simulink library "Blocks_Lib"  (R2019b)
settings: Solver=VariableStepAuto  StartTime=0.0  StopTime=10.0  RelTol=1e-3
libraries: simulink x9, $bdroot x9
(part 2 of 2)

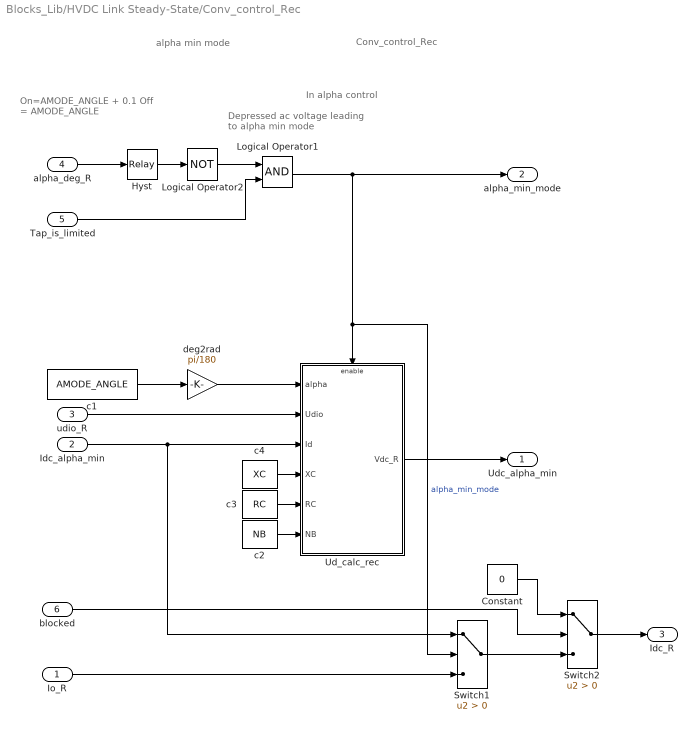
== system Blocks_Lib/HVDC Link Steady-State/Conv_control_Rec ==
  note: Depressed ac voltage
      |  leading to alpha min mode
  note: In alpha control
  note: Conv_control_Rec
  note: On=AMODE_ANGLE + 0.1
      | Off = AMODE_ANGLE
  note: alpha min mode
  Io_R : Inport
  Idc_alpha_min : Inport  Port=2
  udio_R : Inport  Port=3
  alpha_deg_R : Inport  Port=4
  Tap_is_limited : Inport  Port=5
  blocked : Inport  Port=6
  Constant : Constant  Value=0
  Hyst : Relay  OnSwitchValue=AMODE_ANGLE + 0.1  OffSwitchValue=AMODE_ANGLE
  Logical Operator1 : Logic  AllPortsSameDT=off  OutDataTypeStr=boolean
  Logical Operator2 : Logic  Operator=NOT  AllPortsSameDT=off  OutDataTypeStr=boolean
  Switch1 : Switch  Criteria=u2 > Threshold
  Switch2 : Switch  Criteria=u2 > Threshold
  Ud_calc_rec : Subsystem
  c1 : Constant  Value=AMODE_ANGLE
  c2 : Constant  Value=NB
  c3 : Constant  Value=RC
  c4 : Constant  Value=XC
  "deg2rad " : Gain  Gain=pi/180
  Udc_alpha_min : Outport
  alpha_min_mode : Outport  Port=2
  Idc_R : Outport  Port=3
  wires:
  Tap_is_limited/1 -> Logical Operator1/2
  Io_R/1 -> Switch1/3
  Logical Operator1/1 -> alpha_min_mode/1, Ud_calc_rec/Enable, Switch1/2  "alpha_min_mode"
  "deg2rad "/1 -> Ud_calc_rec/1(alpha)
  c1/1 -> "deg2rad "/1
  udio_R/1 -> Ud_calc_rec/2(Udio)
  c3/1 -> Ud_calc_rec/5(RC)
  c4/1 -> Ud_calc_rec/4(XC)
  alpha_deg_R/1 -> Hyst/1
  Ud_calc_rec/1(Vdc_R) -> Udc_alpha_min/1
  Idc_alpha_min/1 -> Ud_calc_rec/3(Id), Switch1/1
  Switch1/1 -> Switch2/3
  Switch2/1 -> Idc_R/1
  Constant/1 -> Switch2/1
  blocked/1 -> Switch2/2
  Hyst/1 -> Logical Operator2/1
  Logical Operator2/1 -> Logical Operator1/1
  c2/1 -> Ud_calc_rec/6(NB)

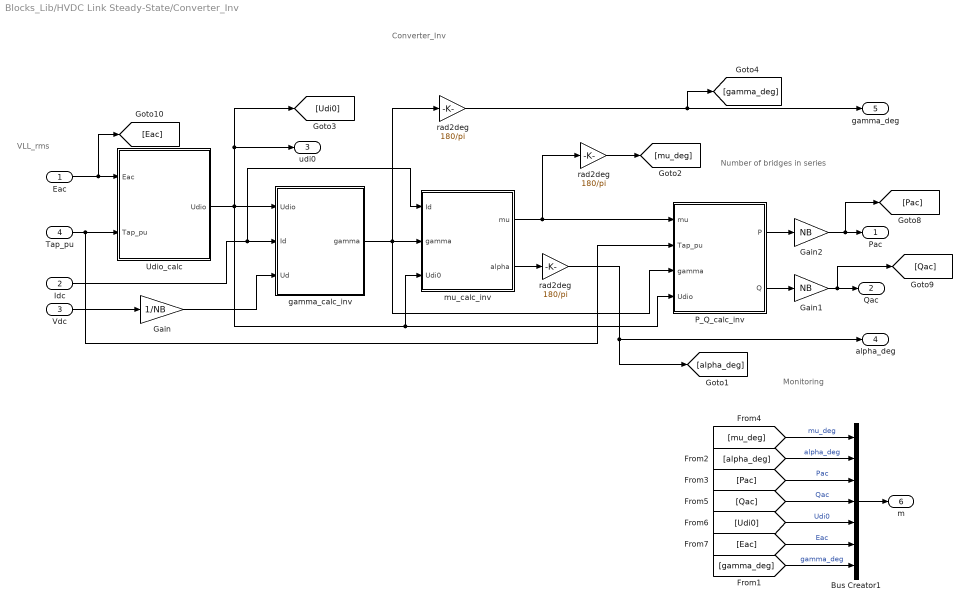
== system Blocks_Lib/HVDC Link Steady-State/Converter_Inv ==
  note: Monitoring
  note: Number of bridges in series
  note: VLL_rms
  note: Converter_Inv
  Eac : Inport
  Idc : Inport  Port=2
  Vdc : Inport  Port=3
  Tap_pu : Inport  Port=4
  Bus Creator1 : BusCreator  Inputs=7
  Gain : Gain  Gain=1/NB
  Gain1 : Gain  Gain=NB
  Gain2 : Gain  Gain=NB
  P_Q_calc_inv : Subsystem
  Udio_calc : Subsystem
  gamma_calc_inv : Subsystem
  mu_calc_inv : Subsystem
  "rad2deg " : Gain  Gain=180/pi
  "rad2deg  " : Gain  Gain=180/pi
  "rad2deg   " : Gain  Gain=180/pi
  Pac : Outport
  Qac : Outport  Port=2
  udi0 : Outport  Port=3
  alpha_deg : Outport  Port=4
  gamma_deg : Outport  Port=5
  m : Outport  Port=6
  wires:
  [Eac] -> Bus Creator1/6  "Eac"
  [gamma_deg] -> Bus Creator1/7  "gamma_deg"
  [Udi0] -> Bus Creator1/5  "Udi0"
  [Qac] -> Bus Creator1/4  "Qac"
  [Pac] -> Bus Creator1/3  "Pac"
  [alpha_deg] -> Bus Creator1/2  "alpha_deg"
  [mu_deg] -> Bus Creator1/1  "mu_deg"
  Bus Creator1/1 -> m/1
  "rad2deg   "/1 -> [alpha_deg], alpha_deg/1
  mu_calc_inv/2(alpha) -> "rad2deg   "/1
  mu_calc_inv/1(mu) -> "rad2deg  "/1, P_Q_calc_inv/1(mu)
  "rad2deg  "/1 -> [mu_deg]
  Gain1/1 -> [Qac], Qac/1
  Gain2/1 -> [Pac], Pac/1
  Gain/1 -> gamma_calc_inv/3(Ud)
  P_Q_calc_inv/1(P) -> Gain2/1
  P_Q_calc_inv/2(Q) -> Gain1/1
  "rad2deg "/1 -> [gamma_deg], gamma_deg/1
  gamma_calc_inv/1(gamma) -> P_Q_calc_inv/3(gamma), mu_calc_inv/2(gamma), "rad2deg "/1
  Vdc/1 -> Gain/1
  Idc/1 -> mu_calc_inv/1(Id), gamma_calc_inv/2(Id)
  Eac/1 -> [Eac], Udio_calc/1(Eac)
  Udio_calc/1(Udio) -> [Udi0], udi0/1, P_Q_calc_inv/4(Udio), mu_calc_inv/3(Udi0), gamma_calc_inv/1(Udio)
  Tap_pu/1 -> P_Q_calc_inv/2(Tap_pu), Udio_calc/2(Tap_pu)

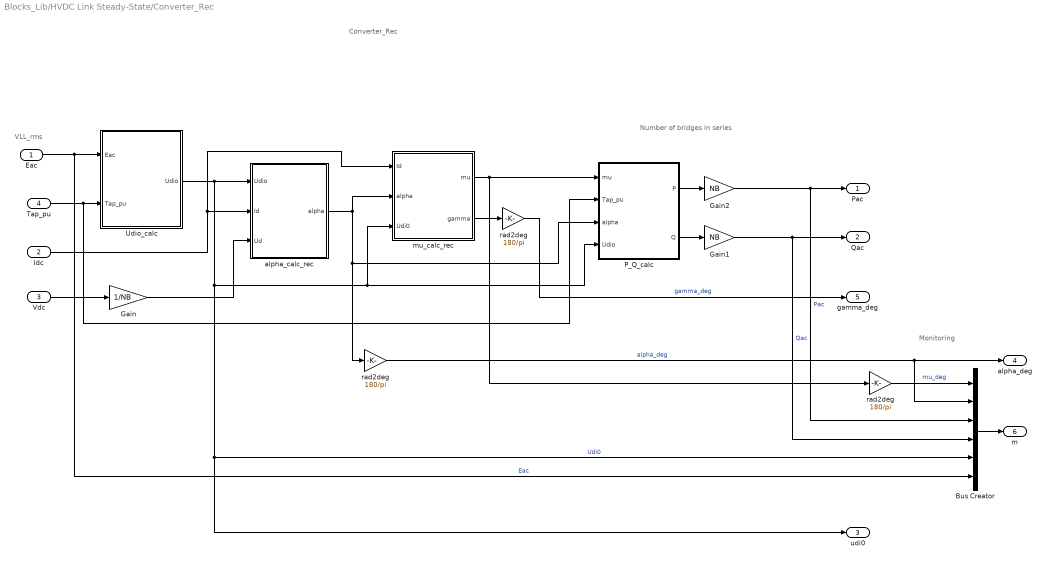
== system Blocks_Lib/HVDC Link Steady-State/Converter_Rec ==
  note: Converter_Rec
  note: VLL_rms
  note: Number of bridges in series
  note: Monitoring
  Eac : Inport
  Idc : Inport  Port=2
  Vdc : Inport  Port=3
  Tap_pu : Inport  Port=4
  Bus Creator : BusCreator  Inputs=6
  Gain : Gain  Gain=1/NB
  Gain1 : Gain  Gain=NB
  Gain2 : Gain  Gain=NB
  P_Q_calc : Subsystem
  Udio_calc : Subsystem
  alpha_calc_rec : Subsystem
  mu_calc_rec : Subsystem
  "rad2deg " : Gain  Gain=180/pi
  "rad2deg  " : Gain  Gain=180/pi
  "rad2deg   " : Gain  Gain=180/pi
  Pac : Outport
  Qac : Outport  Port=2
  udi0 : Outport  Port=3
  alpha_deg : Outport  Port=4
  gamma_deg : Outport  Port=5
  m : Outport  Port=6
  wires:
  Eac/1 -> Udio_calc/1(Eac), Bus Creator/6  "Eac"
  Udio_calc/1(Udio) -> udi0/1, Bus Creator/5, mu_calc_rec/3(Udi0), P_Q_calc/4(Udio), alpha_calc_rec/1(Udio)  "Udi0"
  Gain1/1 -> Bus Creator/4, Qac/1  "Qac"
  Gain2/1 -> Bus Creator/3, Pac/1  "Pac"
  "rad2deg "/1 -> Bus Creator/2, alpha_deg/1  "alpha_deg"
  "rad2deg  "/1 -> Bus Creator/1  "mu_deg"
  Tap_pu/1 -> P_Q_calc/2(Tap_pu), Udio_calc/2(Tap_pu)
  Idc/1 -> alpha_calc_rec/2(Id), mu_calc_rec/1(Id)
  Vdc/1 -> Gain/1
  alpha_calc_rec/1(alpha) -> "rad2deg "/1, P_Q_calc/3(alpha), mu_calc_rec/2(alpha)
  mu_calc_rec/1(mu) -> P_Q_calc/1(mu), "rad2deg  "/1
  mu_calc_rec/2(gamma) -> "rad2deg   "/1
  P_Q_calc/2(Q) -> Gain1/1
  P_Q_calc/1(P) -> Gain2/1
  Gain/1 -> alpha_calc_rec/3(Ud)
  Bus Creator/1 -> m/1
  "rad2deg   "/1 -> gamma_deg/1  "gamma_deg"

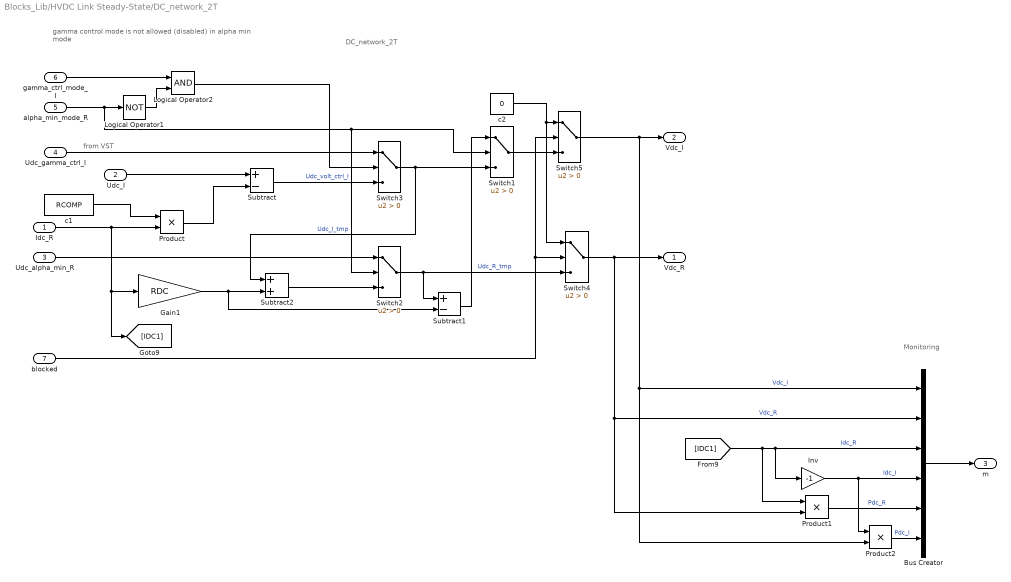
== system Blocks_Lib/HVDC Link Steady-State/DC_network_2T ==
  note: gamma control mode is not allowed (disabled)
      |  in alpha min mode
  note: DC_network_2T
  note: Monitoring
  note: from VST
  Idc_R : Inport
  Udc_I : Inport  Port=2
  Udc_alpha_min_R : Inport  Port=3
  Udc_gamma_ctrl_I : Inport  Port=4
  alpha_min_mode_R : Inport  Port=5
  gamma_ctrl_mode_I : Inport  Port=6
  blocked : Inport  Port=7
  Bus Creator : BusCreator  Inputs=6
  Gain1 : Gain  Gain=RDC
  Inv : Gain  Gain=-1
  Logical Operator1 : Logic  Operator=NOT  AllPortsSameDT=off  OutDataTypeStr=boolean
  Logical Operator2 : Logic  AllPortsSameDT=off  OutDataTypeStr=boolean
  Product : Product  RndMeth=Zero
  Product1 : Product  RndMeth=Zero
  Product2 : Product  RndMeth=Zero
  Subtract : Sum  Inputs=+-
  Subtract1 : Sum  Inputs=+-
  Subtract2 : Sum
  Switch{1..5} (5 alike) : Switch  Criteria=u2 > Threshold
  c1 : Constant  Value=RCOMP
  c2 : Constant  Value=0
  Vdc_R : Outport
  Vdc_I : Outport  Port=2
  m : Outport  Port=3
  wires:
  Product2/1 -> Bus Creator/6  "Pdc_I"
  [IDC1] -> Bus Creator/3, Inv/1, Product1/1  "Idc_R"
  Product1/1 -> Bus Creator/5  "Pdc_R"
  Inv/1 -> Product2/1, Bus Creator/4  "Idc_I"
  Logical Operator2/1 -> Switch3/2
  alpha_min_mode_R/1 -> Switch1/2, Switch2/2, Logical Operator1/1
  Logical Operator1/1 -> Logical Operator2/2
  gamma_ctrl_mode_I/1 -> Logical Operator2/1
  Udc_I/1 -> Subtract/1
  Idc_R/1 -> [IDC1], Gain1/1, Product/2
  Subtract/1 -> Switch3/3  "Udc_volt_ctrl_I"
  Udc_gamma_ctrl_I/1 -> Switch3/1
  Switch3/1 -> Switch1/3, Subtract2/1  "Udc_I_tmp"
  Gain1/1 -> Subtract2/2, Subtract1/2
  Subtract2/1 -> Switch2/3
  Udc_alpha_min_R/1 -> Switch2/1
  Switch2/1 -> Subtract1/1, Switch4/3  "Udc_R_tmp"
  Subtract1/1 -> Switch1/1
  Product/1 -> Subtract/2
  c1/1 -> Product/1
  Bus Creator/1 -> m/1
  Switch5/1 -> Bus Creator/1, Product2/2, Vdc_I/1  "Vdc_I"
  Switch4/1 -> Bus Creator/2, Product1/2, Vdc_R/1  "Vdc_R"
  Switch1/1 -> Switch5/3
  blocked/1 -> Switch4/2, Switch5/2
  c2/1 -> Switch5/1, Switch4/1

== system Blocks_Lib/HVDC Link Steady-State/LF_Soution_Criteria ==
  note: convergence criteria for DC LF solution
  Tap_R : Inport
  Tap_I : Inport  Port=2
  Tap_is_limited_R : Inport  Port=3
  Tap_is_limited_I : Inport  Port=4
  Abs : Abs
  Abs1 : Abs
  Compare To Constant : simulink/Logic and Bit Operations/Compare To Constant  relop=<=  const=1e-6  OutDataTypeStr=uint8
  Compare To Constant1 : simulink/Logic and Bit Operations/Compare To Constant  relop=<=  const=1e-6  OutDataTypeStr=uint8
  Difference : simulink/Discrete/Difference  ICPrevInput=0.0  InputProcessing=Inherited  OutMin=[]  OutMax=[]  OutDataType=fixdt(1, 16)  OutScaling=2^-10  DoSatur=off
  Difference1 : simulink/Discrete/Difference  ICPrevInput=0.0  InputProcessing=Inherited  OutMin=[]  OutMax=[]  OutDataType=fixdt(1, 16)  OutScaling=2^-10  DoSatur=off
  Logical Operator : Logic  AllPortsSameDT=off  OutDataTypeStr=boolean
  Logical Operator1 : Logic  AllPortsSameDT=off  OutDataTypeStr=boolean
  Logical Operator2 : Logic  Operator=NOT  AllPortsSameDT=off  OutDataTypeStr=boolean
  Logical Operator3 : Logic  Operator=OR  AllPortsSameDT=off  OutDataTypeStr=boolean
  Logical Operator4 : Logic  AllPortsSameDT=off  OutDataTypeStr=boolean
  Logical Operator5 : Logic  Operator=OR  AllPortsSameDT=off  OutDataTypeStr=boolean
  Logical Operator6 : Logic  Operator=NOT  AllPortsSameDT=off  OutDataTypeStr=boolean
  Unit Delay1 : UnitDelay  SampleTime=-1  HasFrameUpgradeWarning=on
  Unit Delay2 : UnitDelay  SampleTime=-1  HasFrameUpgradeWarning=on
  converge : Outport
  wires:
  Tap_I/1 -> Difference/1
  Tap_R/1 -> Difference1/1
  Difference1/1 -> Abs1/1
  Abs1/1 -> Compare To Constant1/1
  Abs/1 -> Compare To Constant/1
  Logical Operator/1 -> converge/1
  Difference/1 -> Abs/1
  Compare To Constant/1 -> Logical Operator1/1
  Tap_is_limited_I/1 -> Logical Operator2/1, Unit Delay2/1
  Logical Operator2/1 -> Logical Operator1/2
  Logical Operator1/1 -> Logical Operator3/1
  Logical Operator3/1 -> Logical Operator/2
  Unit Delay2/1 -> Logical Operator3/2
  Compare To Constant1/1 -> Logical Operator4/1
  Logical Operator4/1 -> Logical Operator5/1
  Tap_is_limited_R/1 -> Unit Delay1/1, Logical Operator6/1
  Logical Operator6/1 -> Logical Operator4/2
  Unit Delay1/1 -> Logical Operator5/2
  Logical Operator5/1 -> Logical Operator/1

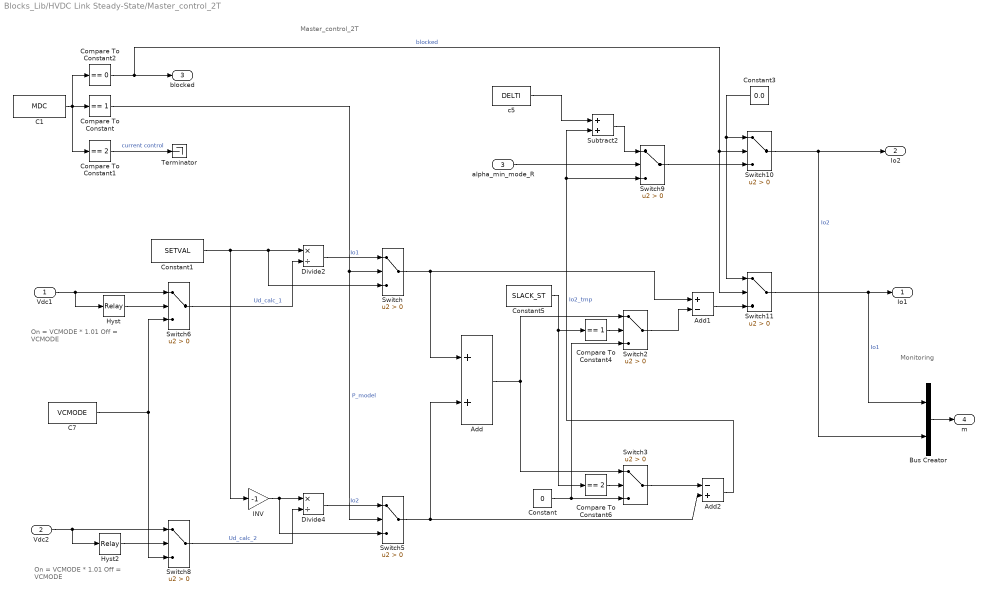
== system Blocks_Lib/HVDC Link Steady-State/Master_control_2T ==
  note: Master_control_2T
  note: On = VCMODE  * 1.01
      | Off = VCMODE
  note: On = VCMODE  * 1.01
      | Off = VCMODE
  note: Monitoring
  Vdc1 : Inport
  Vdc2 : Inport  Port=2
  alpha_min_mode_R : Inport  Port=3
  Add : Sum
  Add1 : Sum  Inputs=+-
  Add2 : Sum  Inputs=-+
  Bus Creator : BusCreator  Inputs=2
  C1 : Constant  Value=MDC
  C7 : Constant  Value=VCMODE
  Compare To Constant : simulink/Logic and Bit Operations/Compare To Constant  relop===  const=1  OutDataTypeStr=uint8  ZeroCross=off
  Compare To Constant1 : simulink/Logic and Bit Operations/Compare To Constant  relop===  const=2  OutDataTypeStr=uint8  ZeroCross=off
  Compare To Constant2 : simulink/Logic and Bit Operations/Compare To Constant  relop===  const=0  OutDataTypeStr=uint8  ZeroCross=off
  Compare To Constant4 : simulink/Logic and Bit Operations/Compare To Constant  relop===  const=1  OutDataTypeStr=uint8
  Compare To Constant6 : simulink/Logic and Bit Operations/Compare To Constant  relop===  const=2  OutDataTypeStr=uint8
  Constant : Constant  Value=0
  Constant1 : Constant  Value=SETVAL
  Constant3 : Constant  Value=0.0
  Constant5 : Constant  Value=SLACK_ST
  Divide2 : Product  Inputs=*/
  Divide4 : Product  Inputs=*/
  Hyst : Relay  OnSwitchValue=VCMODE*1.01  OffSwitchValue=VCMODE
  Hyst2 : Relay  OnSwitchValue=VCMODE*1.01  OffSwitchValue=VCMODE
  INV : Gain  Gain=-1
  Subtract2 : Sum
  Switch{,2..3,5..6,8..11} (9 alike) : Switch  Criteria=u2 > Threshold
  Terminator : Terminator
  c5 : Constant  Value=DELTI
  Io1 : Outport
  Io2 : Outport  Port=2
  blocked : Outport  Port=3
  m : Outport  Port=4
  wires:
  Switch10/1 -> Bus Creator/2, Io2/1  "Io2"
  Add1/1 -> Switch11/3
  Constant3/1 -> Switch11/1, Switch10/1
  Switch9/1 -> Switch10/3
  alpha_min_mode_R/1 -> Switch9/2
  Compare To Constant2/1 -> Switch11/2, Switch10/2, blocked/1  "blocked"
  C1/1 -> Compare To Constant1/1, Compare To Constant/1, Compare To Constant2/1
  Compare To Constant1/1 -> Terminator/1  "current control"
  Add/1 -> Switch2/1, Switch3/1
  Switch2/1 -> Add1/2
  INV/1 -> Divide4/1, Switch5/3
  Constant1/1 -> Divide2/1, Switch/3, INV/1
  Compare To Constant4/1 -> Switch2/2
  Compare To Constant6/1 -> Switch3/2
  Constant/1 -> Switch2/3, Switch3/3
  Constant5/1 -> Compare To Constant6/1, Compare To Constant4/1
  Divide2/1 -> Switch/1  "Io1"
  Divide4/1 -> Switch5/1  "Io2"
  Switch/1 -> Add/1, Add1/1
  Switch5/1 -> Add2/2, Add/2
  Compare To Constant/1 -> Switch/2, Switch5/2  "P_model"
  Switch3/1 -> Add2/1
  Hyst/1 -> Switch6/2
  C7/1 -> Switch6/3, Switch8/3
  Vdc1/1 -> Switch6/1, Hyst/1
  Hyst2/1 -> Switch8/2
  Vdc2/1 -> Switch8/1, Hyst2/1
  Switch6/1 -> Divide2/2  "Ud_calc_1"
  Switch8/1 -> Divide4/2  "Ud_calc_2"
  Bus Creator/1 -> m/1
  Add2/1 -> Subtract2/2, Switch9/3  "Io2_tmp"
  c5/1 -> Subtract2/1
  Subtract2/1 -> Switch9/1
  Switch11/1 -> Bus Creator/1, Io1/1  "Io1"

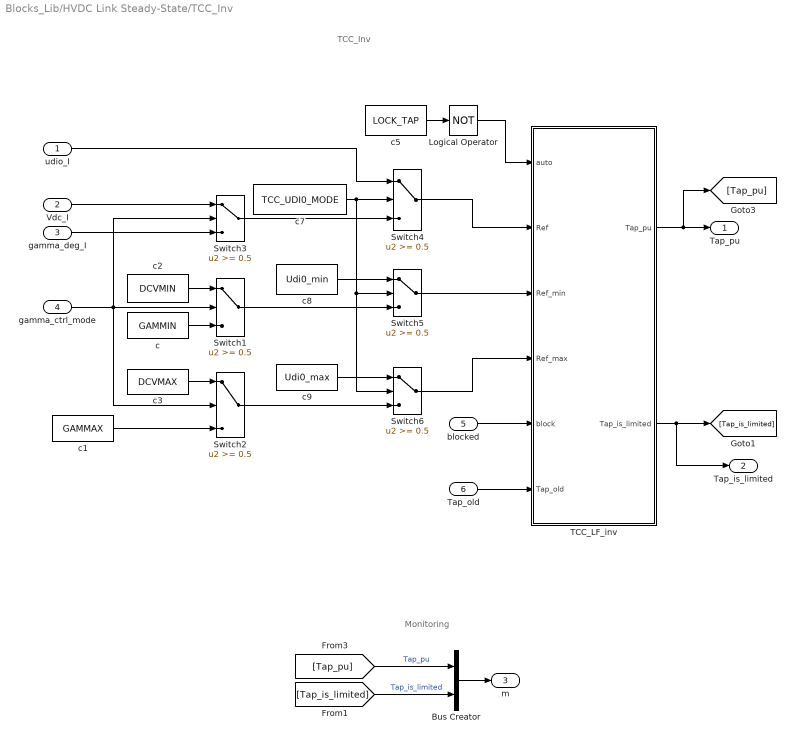
== system Blocks_Lib/HVDC Link Steady-State/TCC_Inv ==
  note: Monitoring
  note: TCC_Inv
  udio_I : Inport
  Vdc_I : Inport  Port=2
  gamma_deg_I : Inport  Port=3
  gamma_ctrl_mode : Inport  Port=4
  blocked : Inport  Port=5
  Tap_old : Inport  Port=6
  Bus Creator : BusCreator  Inputs=2
  Logical Operator : Logic  Operator=NOT  AllPortsSameDT=off  OutDataTypeStr=boolean
  Switch{1..6} (6 alike) : Switch  Threshold=0.5
  TCC_LF_inv : Subsystem
  c : Constant  Value=GAMMIN
  c1 : Constant  Value=GAMMAX
  c2 : Constant  Value=DCVMIN
  c3 : Constant  Value=DCVMAX
  c5 : Constant  Value=LOCK_TAP
  c7 : Constant  Value=TCC_UDI0_MODE
  c8 : Constant  Value=Udi0_min
  c9 : Constant  Value=Udi0_max
  Tap_pu : Outport
  Tap_is_limited : Outport  Port=2
  m : Outport  Port=3
  wires:
  [Tap_is_limited] -> Bus Creator/2  "Tap_is_limited"
  [Tap_pu] -> Bus Creator/1  "Tap_pu"
  Bus Creator/1 -> m/1
  Vdc_I/1 -> Switch3/1
  c2/1 -> Switch1/1
  c3/1 -> Switch2/1
  gamma_deg_I/1 -> Switch3/3
  c1/1 -> Switch2/3
  c/1 -> Switch1/3
  gamma_ctrl_mode/1 -> Switch3/2, Switch2/2, Switch1/2
  blocked/1 -> TCC_LF_inv/5(block)
  c5/1 -> Logical Operator/1
  Logical Operator/1 -> TCC_LF_inv/1(auto)
  udio_I/1 -> Switch4/1
  c7/1 -> Switch4/2, Switch5/2, Switch6/2
  c8/1 -> Switch5/1
  c9/1 -> Switch6/1
  Switch3/1 -> Switch4/3
  Switch1/1 -> Switch5/3
  Switch2/1 -> Switch6/3
  Switch4/1 -> TCC_LF_inv/2(Ref)
  Switch5/1 -> TCC_LF_inv/3(Ref_min)
  Switch6/1 -> TCC_LF_inv/4(Ref_max)
  Tap_old/1 -> TCC_LF_inv/6(Tap_old)
  TCC_LF_inv/2(Tap_is_limited) -> [Tap_is_limited], Tap_is_limited/1
  TCC_LF_inv/1(Tap_pu) -> [Tap_pu], Tap_pu/1

== system Blocks_Lib/HVDC Link Steady-State/TCC_Rec ==
  note: TCC_Rec
  note: Monitoring
  udio_R : Inport
  alpha_deg_R : Inport  Port=2
  blocked : Inport  Port=3
  Tap_old : Inport  Port=4
  Bus Creator : BusCreator  Inputs=2
  Logical Operator : Logic  Operator=NOT  AllPortsSameDT=off  OutDataTypeStr=boolean
  Switch4 : Switch  Threshold=0.5
  Switch5 : Switch  Threshold=0.5
  Switch6 : Switch  Threshold=0.5
  TCC_LF : Subsystem
  c1 : Constant  Value=ALFMAX
  c2 : Constant  Value=ALFMIN
  c5 : Constant  Value=LOCK_TAP
  c7 : Constant  Value=TCC_UDI0_MODE
  c8 : Constant  Value=Udi0_min
  c9 : Constant  Value=Udi0_max
  Tap_pu : Outport
  Tap_is_limited : Outport  Port=2
  m : Outport  Port=3
  wires:
  Tap_old/1 -> TCC_LF/6(Tap_old)
  blocked/1 -> TCC_LF/5(block)
  c5/1 -> Logical Operator/1
  Logical Operator/1 -> TCC_LF/1(auto)
  udio_R/1 -> Switch4/1
  c7/1 -> Switch6/2, Switch5/2, Switch4/2
  c8/1 -> Switch5/1
  c9/1 -> Switch6/1
  alpha_deg_R/1 -> Switch4/3
  c1/1 -> Switch6/3
  Switch4/1 -> TCC_LF/2(Ref)
  Switch5/1 -> TCC_LF/3(Ref_min)
  Switch6/1 -> TCC_LF/4(Ref_max)
  c2/1 -> Switch5/3
  Bus Creator/1 -> m/1
  TCC_LF/1(Tap_pu) -> Bus Creator/1, Tap_pu/1  "Tap_pu"
  TCC_LF/2(Tap_is_limited) -> Bus Creator/2, Tap_is_limited/1  "Tap_is_limited"

== system Blocks_Lib/HVDC Link Steady-State/Conv_control_Inv_vst/Ud_calc_inv ==
  note: Equivalent commtating resistance
  note: 3/pi
  note: Udio * cos(gamma)
  note: Ud_calc_inv
  note: Transformer windings & Thyristor
      |  resistance drop
  gamma : Inport
  Udio : Inport  Port=2
  Id : Inport  Port=3
  XC : Inport  Port=4
  RC : Inport  Port=5
  NB : Inport  Port=6
  Enable (held) : EnablePort  PropagateVarSize=During execution
  Gain1 : Gain  Gain=2
  Gain2 : Gain  Gain=3/pi
  Product{1..4} (4 alike) : Product  RndMeth=Zero
  Subtract : Sum  Inputs=+-+
  Trigonometric Function : Trigonometry  Operator=cos
  Vdc_I : Outport
  wires:
  gamma/1 -> Trigonometric Function/1
  Trigonometric Function/1 -> Product1/2
  Udio/1 -> Product1/1
  Product1/1 -> Subtract/1  "udio_cos_gamma"
  Id/1 -> Product2/1, Product4/1
  Product2/1 -> Subtract/2  "RcId"
  Gain2/1 -> Product2/2
  RC/1 -> Gain1/1
  Gain1/1 -> Product4/2
  Product4/1 -> Subtract/3
  XC/1 -> Gain2/1
  Subtract/1 -> Product3/1
  Product3/1 -> Vdc_I/1
  NB/1 -> Product3/2

== system Blocks_Lib/HVDC Link Steady-State/Conv_control_Rec/Ud_calc_rec ==
  note: Equivalent commtating resistance
  note: 3/pi
  note: Udio * cos(alpha)
  note: Ud_calc_rec
  note: Transformer windings & Thyristor
      |  resistance drop
  alpha : Inport
  Udio : Inport  Port=2
  Id : Inport  Port=3
  XC : Inport  Port=4
  RC : Inport  Port=5
  NB : Inport  Port=6
  Enable (held) : EnablePort  PropagateVarSize=During execution
  Gain1 : Gain  Gain=2
  Gain2 : Gain  Gain=3/pi
  Product{1..4} (4 alike) : Product  RndMeth=Zero
  Subtract : Sum  Inputs=+--
  Trigonometric Function : Trigonometry  Operator=cos
  Vdc_R : Outport
  wires:
  alpha/1 -> Trigonometric Function/1
  Trigonometric Function/1 -> Product1/2
  Udio/1 -> Product1/1
  Product1/1 -> Subtract/1  "udio_cos_alpha"
  Id/1 -> Product2/1, Product4/1
  Product2/1 -> Subtract/2  "RcId"
  Gain2/1 -> Product2/2
  RC/1 -> Gain1/1
  Gain1/1 -> Product4/2
  Product4/1 -> Subtract/3
  XC/1 -> Gain2/1
  Subtract/1 -> Product3/1
  Product3/1 -> Vdc_R/1
  NB/1 -> Product3/2

== system Blocks_Lib/HVDC Link Steady-State/Converter_Inv/P_Q_calc_inv ==
  note: Negative in inverter
      |  (gamma)
  mu : Inport
  Tap_pu : Inport  Port=2
  gamma : Inport  Port=3
  Udio : Inport  Port=4
  "Avoid zero " : Saturate  UpperLimit=inf  LowerLimit=eps
  Gain1 : Gain  Gain=NB
  Gain2 : Gain  Gain=NB
  Gain3 : Gain  Gain=-1
  Id_Iq_Pq_calc : Subsystem
  Terminator : Terminator
  Terminator1 : Terminator
  P : Outport
  Q : Outport  Port=2
  wires:
  Gain1/1 -> Terminator1/1
  Gain2/1 -> Terminator/1
  Id_Iq_Pq_calc/4(P_q) -> Q/1
  Id_Iq_Pq_calc/3(P_d) -> Gain3/1
  Udio/1 -> Id_Iq_Pq_calc/1(Udio)
  "Avoid zero "/1 -> Id_Iq_Pq_calc/2(Tap_pu)
  Tap_pu/1 -> "Avoid zero "/1
  mu/1 -> Id_Iq_Pq_calc/3(mu)
  gamma/1 -> Id_Iq_Pq_calc/4(angle)
  Id_Iq_Pq_calc/1(I_d) -> Gain2/1
  Id_Iq_Pq_calc/2(I_q) -> Gain1/1
  Gain3/1 -> P/1

== system Blocks_Lib/HVDC Link Steady-State/Converter_Inv/Udio_calc ==
  note: Udio_calc
  note: 3*sqrt(2)/pi * Usec_nom/Uprim_nom
  note: VLL_rms
  Eac : Inport
  Tap_pu : Inport  Port=2
  "Avoid zero " : Saturate  UpperLimit=inf  LowerLimit=eps
  Divide3 : Product  Inputs=*/
  k : Gain  Gain=(3*sqrt(2)/pi) * TR
  Udio : Outport
  wires:
  Divide3/1 -> Udio/1
  Tap_pu/1 -> "Avoid zero "/1
  "Avoid zero "/1 -> Divide3/2
  Eac/1 -> k/1
  k/1 -> Divide3/1

== system Blocks_Lib/HVDC Link Steady-State/Converter_Inv/gamma_calc_inv ==
  note: Equivalent commtating resistance (Rc)
  note: 3/pi
  note: gamma_calc_inv
  note: Transformer windings resistance drop
  Udio : Inport
  Id : Inport  Port=2
  Ud : Inport  Port=3
  Avoid zero : Saturate  UpperLimit=inf  LowerLimit=eps
  Divide : Product  Inputs=*/
  Gain1 : Gain  Gain=2
  Gain2 : Gain  Gain=3/pi
  Min:-1 Max:1 : Saturate  UpperLimit=1.0  LowerLimit=-1.0
  Product2 : Product  RndMeth=Zero
  Product4 : Product  RndMeth=Zero
  Subtract : Sum  Inputs=++-
  Trigonometric Function1 : Trigonometry  Operator=acos
  c : Constant  Value=XC
  c3 : Constant  Value=RC
  gamma : Outport
  wires:
  Id/1 -> Product2/1, Product4/1
  Product2/1 -> Subtract/2  "RcId"
  Gain2/1 -> Product2/2  "Rc"
  Product4/1 -> Subtract/3
  Ud/1 -> Subtract/1
  Subtract/1 -> Divide/1
  Udio/1 -> Avoid zero/1
  Avoid zero/1 -> Divide/2
  Divide/1 -> Min:-1 Max:1/1
  c3/1 -> Gain1/1
  Gain1/1 -> Product4/2
  Trigonometric Function1/1 -> gamma/1
  c/1 -> Gain2/1
  Min:-1 Max:1/1 -> Trigonometric Function1/1

== system Blocks_Lib/HVDC Link Steady-State/Converter_Inv/mu_calc_inv ==
  note: Uac_sec_LL_rms / sqrt(2)
  note: pi/6
  note: mu_calc_inv
  note: mu = arcos( cos (gamma - 2 (Xc*3/pi*Id/ Udio)) - gamma
  note: alpha = pi - gamma - mu
  Id : Inport
  gamma : Inport  Port=2
  Udi0 : Inport  Port=3
  Avoid zero : Saturate  UpperLimit=inf  LowerLimit=eps
  Constant : Constant  Value=pi
  Divide1 : Product  Inputs=*/
  Divide2 : Product  Inputs=*/
  Gain2 : Gain  Gain=pi/6
  Min=-1 Max=1 : Saturate  UpperLimit=1  LowerLimit=-1
  Subtract1 : Sum  Inputs=+-
  Subtract2 : Sum  Inputs=+-
  Subtract3 : Sum  Inputs=--+
  Trigonometric Function : Trigonometry  Operator=acos
  Trigonometric Function1 : Trigonometry  Operator=cos
  c : Constant  Value=XC
  mu : Outport
  alpha : Outport  Port=2
  wires:
  Trigonometric Function1/1 -> Subtract1/1
  Subtract3/1 -> alpha/1
  Divide2/1 -> Avoid zero/1  "Is2"
  Gain2/1 -> Divide2/1
  Udi0/1 -> Gain2/1
  Subtract2/1 -> mu/1, Subtract3/1
  gamma/1 -> Trigonometric Function1/1, Subtract3/2, Subtract2/2
  Trigonometric Function/1 -> Subtract2/1
  Subtract1/1 -> Min=-1 Max=1/1
  Divide1/1 -> Subtract1/2
  Avoid zero/1 -> Divide1/2
  Id/1 -> Divide1/1
  c/1 -> Divide2/2
  Min=-1 Max=1/1 -> Trigonometric Function/1
  Constant/1 -> Subtract3/3

== system Blocks_Lib/HVDC Link Steady-State/Converter_Rec/P_Q_calc ==
  note: P_Q_calc
  mu : Inport
  Tap_pu : Inport  Port=2
  alpha : Inport  Port=3
  Udio : Inport  Port=4
  "Avoid zero " : Saturate  UpperLimit=inf  LowerLimit=eps
  Gain1 : Gain  Gain=NB
  Gain2 : Gain  Gain=NB
  Id_Iq_Pq_calc : Subsystem
  Terminator : Terminator
  Terminator1 : Terminator
  P : Outport
  Q : Outport  Port=2
  wires:
  Id_Iq_Pq_calc/2(I_q) -> Gain1/1
  Id_Iq_Pq_calc/1(I_d) -> Gain2/1
  alpha/1 -> Id_Iq_Pq_calc/4(angle)
  mu/1 -> Id_Iq_Pq_calc/3(mu)
  Tap_pu/1 -> "Avoid zero "/1
  "Avoid zero "/1 -> Id_Iq_Pq_calc/2(Tap_pu)
  Udio/1 -> Id_Iq_Pq_calc/1(Udio)
  Id_Iq_Pq_calc/3(P_d) -> P/1
  Id_Iq_Pq_calc/4(P_q) -> Q/1
  Gain2/1 -> Terminator/1
  Gain1/1 -> Terminator1/1

== system Blocks_Lib/HVDC Link Steady-State/Converter_Rec/Udio_calc ==
  note: VLL_rms
  note: 3*sqrt(2)/pi * Usec_nom/Uprim_nom
  note: Udio_calc
  Eac : Inport
  Tap_pu : Inport  Port=2
  "Avoid zero " : Saturate  UpperLimit=inf  LowerLimit=eps
  Divide3 : Product  Inputs=*/
  k : Gain  Gain=(3*sqrt(2)/pi) * TR
  Udio : Outport
  wires:
  k/1 -> Divide3/1
  Eac/1 -> k/1
  "Avoid zero "/1 -> Divide3/2
  Tap_pu/1 -> "Avoid zero "/1
  Divide3/1 -> Udio/1

== system Blocks_Lib/HVDC Link Steady-State/Converter_Rec/alpha_calc_rec ==
  note: Equivalent commtating resistance (Rc)
  note: 3/pi
  note: alpha_calc_rec
  note: Transformer windings resistance drop
  Udio : Inport
  Id : Inport  Port=2
  Ud : Inport  Port=3
  Avoid zero : Saturate  UpperLimit=inf  LowerLimit=eps
  Divide : Product  Inputs=*/
  Gain1 : Gain  Gain=2
  Gain2 : Gain  Gain=3/pi
  Min:-1 Max:1 : Saturate  UpperLimit=1.0  LowerLimit=-1.0
  Product2 : Product  RndMeth=Zero
  Product4 : Product  RndMeth=Zero
  Subtract : Sum  Inputs=+++
  Trigonometric Function1 : Trigonometry  Operator=acos
  c : Constant  Value=XC
  c3 : Constant  Value=RC
  alpha : Outport
  wires:
  c/1 -> Gain2/1
  Id/1 -> Product2/1, Product4/1
  Product2/1 -> Subtract/2  "RcId"
  Gain2/1 -> Product2/2  "Rc"
  Product4/1 -> Subtract/3
  Ud/1 -> Subtract/1
  Subtract/1 -> Divide/1
  Udio/1 -> Avoid zero/1
  Avoid zero/1 -> Divide/2
  Divide/1 -> Min:-1 Max:1/1
  Gain1/1 -> Product4/2
  Trigonometric Function1/1 -> alpha/1
  c3/1 -> Gain1/1
  Min:-1 Max:1/1 -> Trigonometric Function1/1

== system Blocks_Lib/HVDC Link Steady-State/Converter_Rec/mu_calc_rec ==
  note: gamma = pi - alpha - mu
  note: mu = arcos( cos (alpha) - 2 (Xc*3/pi*Id/ Udio)) - alpha
  note: mu_calc
  note: pi/6
  note: Uac_sec_LL_rms / sqrt(2)
  Id : Inport
  alpha : Inport  Port=2
  Udi0 : Inport  Port=3
  Avoid zero : Saturate  UpperLimit=inf  LowerLimit=eps
  Constant : Constant  Value=pi
  Divide1 : Product  Inputs=*/
  Divide2 : Product  Inputs=*/
  Gain2 : Gain  Gain=pi/6
  Min=-1 Max=1 : Saturate  UpperLimit=1  LowerLimit=-1
  Subtract1 : Sum  Inputs=+-
  Subtract2 : Sum  Inputs=+-
  Subtract3 : Sum  Inputs=--+
  Trigonometric Function : Trigonometry  Operator=acos
  Trigonometric Function1 : Trigonometry  Operator=cos
  c : Constant  Value=XC
  mu : Outport
  gamma : Outport  Port=2
  wires:
  Constant/1 -> Subtract3/3
  Min=-1 Max=1/1 -> Trigonometric Function/1
  c/1 -> Divide2/2
  Id/1 -> Divide1/1
  Avoid zero/1 -> Divide1/2
  Divide1/1 -> Subtract1/2
  Subtract1/1 -> Min=-1 Max=1/1
  Trigonometric Function/1 -> Subtract2/1
  alpha/1 -> Subtract2/2, Subtract3/2, Trigonometric Function1/1
  Subtract2/1 -> Subtract3/1, mu/1
  Udi0/1 -> Gain2/1
  Gain2/1 -> Divide2/1
  Divide2/1 -> Avoid zero/1  "Is2"
  Subtract3/1 -> gamma/1
  Trigonometric Function1/1 -> Subtract1/1

== system Blocks_Lib/HVDC Link Steady-State/TCC_Inv/TCC_LF_inv ==
  note: Automatic mode
  note: Tap step (pu)
  auto : Inport
  Ref : Inport  Port=2
  Ref_min : Inport  Port=3
  Ref_max : Inport  Port=4
  block : Inport  Port=5
  Tap_old : Inport  Port=6
  (TSTP) : Quantizer  QuantizationInterval=TSTP
  Add : Sum  Inputs=+-+
  Logical Operator : Logic  Inputs=3  AllPortsSameDT=off  OutDataTypeStr=boolean
  Logical Operator1 : Logic  Operator=NOT  AllPortsSameDT=off  OutDataTypeStr=boolean
  Logical Operator2 : Logic  Inputs=3  AllPortsSameDT=off  OutDataTypeStr=boolean
  Max=TAPMX Min=TAPMN : Saturate  UpperLimit=TAPMX  LowerLimit=TAPMN
  Relational Operator : RelationalOperator  Operator=<  OutDataTypeStr=boolean  RndMeth=Nearest
  Relational Operator1 : RelationalOperator  Operator=>  OutDataTypeStr=boolean  RndMeth=Nearest
  Relational Operator2 : RelationalOperator  Operator=~=  OutDataTypeStr=boolean  RndMeth=Nearest
  Switch : Switch  Threshold=0.5
  Switch1 : Switch  Threshold=0.5
  Tap_step : Constant  Value=TSTP
  zero : Constant  Value=0
  Tap_pu : Outport
  Tap_is_limited : Outport  Port=2
  wires:
  Tap_old/1 -> (TSTP)/1
  (TSTP)/1 -> Add/1
  Ref_min/1 -> Relational Operator/2
  Switch1/1 -> Add/3
  Logical Operator2/1 -> Switch1/2
  Ref/1 -> Relational Operator/1, Relational Operator1/1
  Relational Operator1/1 -> Logical Operator2/2  "inc_Np"
  Relational Operator/1 -> Logical Operator/2  "dec_Np"
  Ref_max/1 -> Relational Operator1/2
  Logical Operator1/1 -> Logical Operator2/1, Logical Operator/1
  block/1 -> Logical Operator1/1
  zero/1 -> Switch/3, Switch1/3
  Tap_step/1 -> Switch/1, Switch1/1
  Add/1 -> Relational Operator2/2, Max=TAPMX Min=TAPMN/1
  auto/1 -> Logical Operator/3, Logical Operator2/3
  Switch/1 -> Add/2
  Max=TAPMX Min=TAPMN/1 -> Relational Operator2/1, Tap_pu/1
  Relational Operator2/1 -> Tap_is_limited/1
  Logical Operator/1 -> Switch/2

== system Blocks_Lib/HVDC Link Steady-State/TCC_Rec/TCC_LF ==
  note: Automatic mode
  note: Tap step (pu)
  auto : Inport
  Ref : Inport  Port=2
  Ref_min : Inport  Port=3
  Ref_max : Inport  Port=4
  block : Inport  Port=5
  Tap_old : Inport  Port=6
  (TSTP) : Quantizer  QuantizationInterval=TSTP
  Add : Sum  Inputs=+-+
  Logical Operator : Logic  Inputs=3  AllPortsSameDT=off  OutDataTypeStr=boolean
  Logical Operator1 : Logic  Operator=NOT  AllPortsSameDT=off  OutDataTypeStr=boolean
  Logical Operator2 : Logic  Inputs=3  AllPortsSameDT=off  OutDataTypeStr=boolean
  Max=TAPMX Min=TAPMN : Saturate  UpperLimit=TAPMX  LowerLimit=TAPMN
  Relational Operator : RelationalOperator  Operator=<  OutDataTypeStr=boolean  RndMeth=Nearest
  Relational Operator1 : RelationalOperator  Operator=>  OutDataTypeStr=boolean  RndMeth=Nearest
  Relational Operator2 : RelationalOperator  Operator=~=  OutDataTypeStr=boolean  RndMeth=Nearest
  Switch : Switch  Threshold=0.5
  Switch1 : Switch  Threshold=0.5
  Tap_step : Constant  Value=TSTP
  zero : Constant  Value=0
  Tap_pu : Outport
  Tap_is_limited : Outport  Port=2
  wires:
  Tap_old/1 -> (TSTP)/1
  (TSTP)/1 -> Add/1
  Ref_min/1 -> Relational Operator/2
  Logical Operator/1 -> Switch/2
  Switch1/1 -> Add/3
  Logical Operator2/1 -> Switch1/2
  Ref/1 -> Relational Operator/1, Relational Operator1/1
  Relational Operator1/1 -> Logical Operator2/2  "inc_Np"
  Relational Operator/1 -> Logical Operator/2  "dec_Np"
  Ref_max/1 -> Relational Operator1/2
  Logical Operator1/1 -> Logical Operator/1, Logical Operator2/1
  block/1 -> Logical Operator1/1
  zero/1 -> Switch/3, Switch1/3
  Tap_step/1 -> Switch/1, Switch1/1
  Add/1 -> Relational Operator2/2, Max=TAPMX Min=TAPMN/1
  auto/1 -> Logical Operator/3, Logical Operator2/3
  Switch/1 -> Add/2
  Max=TAPMX Min=TAPMN/1 -> Relational Operator2/1, Tap_pu/1
  Relational Operator2/1 -> Tap_is_limited/1

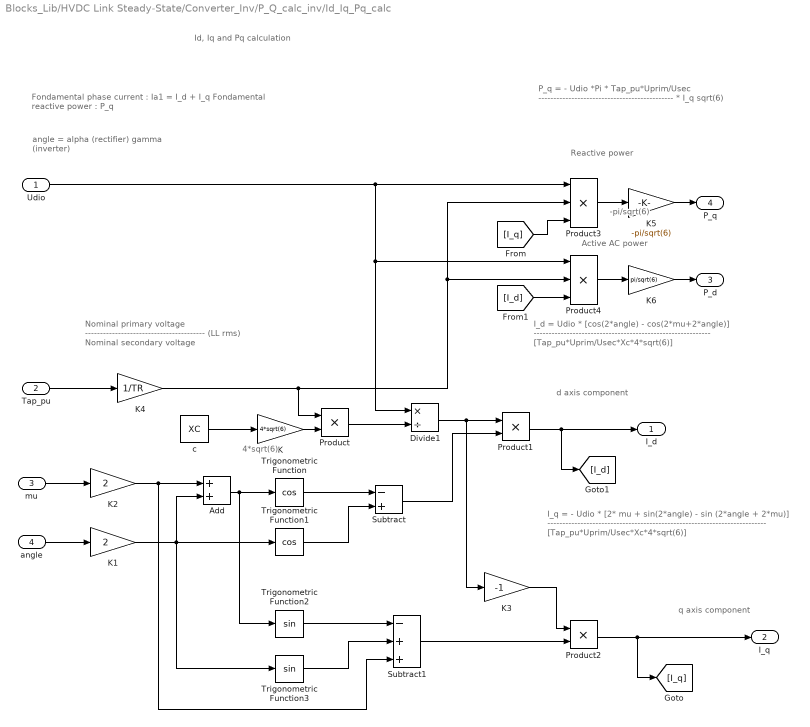
== system Blocks_Lib/HVDC Link Steady-State/Converter_Inv/P_Q_calc_inv/Id_Iq_Pq_calc ==
  note: Active AC power
  note: angle = alpha (rectifier)
      |               gamma (inverter)
  note: P_q =  - Udio *Pi * Tap_pu*Uprim/Usec
      |            --------------------------------------------- * I_q
      |                                sqrt(6)
  note: Reactive power
  note: -pi/sqrt(6)
  note: Id, Iq and Pq calculation
  note: q axis component
  note: d axis component
  note: Fondamental phase current :  Ia1 = I_d + I_q
      | Fondamental reactive power : P_q
  note: I_q = - Udio * [2* mu + sin(2*angle) - sin (2*angle + 2*mu)]
      |           -------------------------------------------------------------------------
      |                        [Tap_pu*Uprim/Usec*Xc*4*sqrt(6)]
  note: Nominal primary voltage
      | ----------------------------------------     (LL rms)
      | Nominal secondary voltage
  note: I_d = Udio * [cos(2*angle) - cos(2*mu+2*angle)]
      |           -----------------------------------------------------------
      |                 [Tap_pu*Uprim/Usec*Xc*4*sqrt(6)]
  note: 4*sqrt(6)
  Udio : Inport
  Tap_pu : Inport  Port=2
  mu : Inport  Port=3
  angle : Inport  Port=4
  Add : Sum
  Divide1 : Product  Inputs=*/
  K : Gain  Gain=4*sqrt(6)
  K1 : Gain  Gain=2
  K2 : Gain  Gain=2
  K3 : Gain  Gain=-1
  K4 : Gain  Gain=1/TR
  K5 : Gain  Gain=-pi/sqrt(6)
  K6 : Gain  Gain=pi/sqrt(6)
  Product : Product  RndMeth=Zero
  Product1 : Product  RndMeth=Zero
  Product2 : Product  RndMeth=Zero
  Product3 : Product  Inputs=3  RndMeth=Zero
  Product4 : Product  Inputs=3  RndMeth=Zero
  Subtract : Sum  Inputs=-+
  Subtract1 : Sum  Inputs=-++
  Trigonometric Function : Trigonometry  Operator=cos
  Trigonometric Function1 : Trigonometry  Operator=cos
  Trigonometric Function2 : Trigonometry
  Trigonometric Function3 : Trigonometry
  c : Constant  Value=XC
  I_d : Outport
  I_q : Outport  Port=2
  P_d : Outport  Port=3
  P_q : Outport  Port=4
  wires:
  K6/1 -> P_d/1
  Product4/1 -> K6/1
  [I_d] -> Product4/3
  K5/1 -> P_q/1
  Product3/1 -> K5/1
  K4/1 -> Product4/2, Product3/2, Product/1
  K3/1 -> Product2/1
  c/1 -> K/1
  K/1 -> Product/2
  Product/1 -> Divide1/2
  Udio/1 -> Product4/1, Divide1/1, Product3/1
  Tap_pu/1 -> K4/1
  angle/1 -> K1/1
  K1/1 -> Add/2, Trigonometric Function1/1, Trigonometric Function3/1
  mu/1 -> K2/1
  K2/1 -> Add/1, Subtract1/3
  Add/1 -> Trigonometric Function/1, Trigonometric Function2/1
  Trigonometric Function/1 -> Subtract/1
  Trigonometric Function1/1 -> Subtract/2
  Divide1/1 -> K3/1, Product1/1
  Subtract/1 -> Product1/2
  Product1/1 -> [I_d], I_d/1
  Trigonometric Function2/1 -> Subtract1/1
  Trigonometric Function3/1 -> Subtract1/2
  Subtract1/1 -> Product2/2
  Product2/1 -> [I_q], I_q/1
  [I_q] -> Product3/3

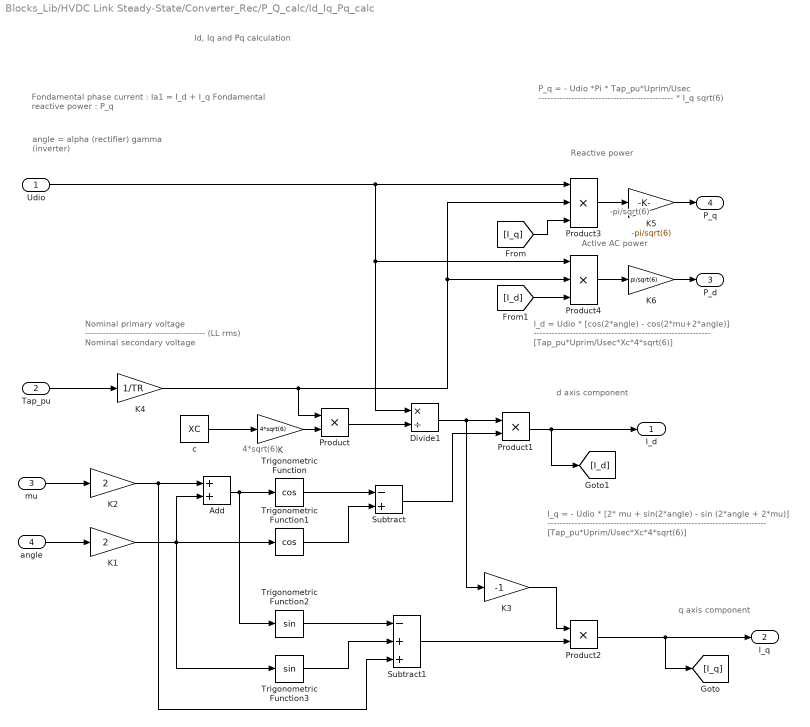
== system Blocks_Lib/HVDC Link Steady-State/Converter_Rec/P_Q_calc/Id_Iq_Pq_calc ==
  note: 4*sqrt(6)
  note: I_d = Udio * [cos(2*angle) - cos(2*mu+2*angle)]
      |           -----------------------------------------------------------
      |                 [Tap_pu*Uprim/Usec*Xc*4*sqrt(6)]
  note: Nominal primary voltage
      | ----------------------------------------     (LL rms)
      | Nominal secondary voltage
  note: I_q = - Udio * [2* mu + sin(2*angle) - sin (2*angle + 2*mu)]
      |           -------------------------------------------------------------------------
      |                        [Tap_pu*Uprim/Usec*Xc*4*sqrt(6)]
  note: Fondamental phase current :  Ia1 = I_d + I_q
      | Fondamental reactive power : P_q
  note: d axis component
  note: q axis component
  note: Id, Iq and Pq calculation
  note: -pi/sqrt(6)
  note: Reactive power
  note: P_q =  - Udio *Pi * Tap_pu*Uprim/Usec
      |            --------------------------------------------- * I_q
      |                                sqrt(6)
  note: angle = alpha (rectifier)
      |               gamma (inverter)
  note: Active AC power
  Udio : Inport
  Tap_pu : Inport  Port=2
  mu : Inport  Port=3
  angle : Inport  Port=4
  Add : Sum
  Divide1 : Product  Inputs=*/
  K : Gain  Gain=4*sqrt(6)
  K1 : Gain  Gain=2
  K2 : Gain  Gain=2
  K3 : Gain  Gain=-1
  K4 : Gain  Gain=1/TR
  K5 : Gain  Gain=-pi/sqrt(6)
  K6 : Gain  Gain=pi/sqrt(6)
  Product : Product  RndMeth=Zero
  Product1 : Product  RndMeth=Zero
  Product2 : Product  RndMeth=Zero
  Product3 : Product  Inputs=3  RndMeth=Zero
  Product4 : Product  Inputs=3  RndMeth=Zero
  Subtract : Sum  Inputs=-+
  Subtract1 : Sum  Inputs=-++
  Trigonometric Function : Trigonometry  Operator=cos
  Trigonometric Function1 : Trigonometry  Operator=cos
  Trigonometric Function2 : Trigonometry
  Trigonometric Function3 : Trigonometry
  c : Constant  Value=XC
  I_d : Outport
  I_q : Outport  Port=2
  P_d : Outport  Port=3
  P_q : Outport  Port=4
  wires:
  [I_q] -> Product3/3
  Product2/1 -> [I_q], I_q/1
  Subtract1/1 -> Product2/2
  Trigonometric Function3/1 -> Subtract1/2
  Trigonometric Function2/1 -> Subtract1/1
  Product1/1 -> [I_d], I_d/1
  Subtract/1 -> Product1/2
  Divide1/1 -> Product1/1, K3/1
  Trigonometric Function1/1 -> Subtract/2
  Trigonometric Function/1 -> Subtract/1
  Add/1 -> Trigonometric Function2/1, Trigonometric Function/1
  K2/1 -> Subtract1/3, Add/1
  mu/1 -> K2/1
  K1/1 -> Trigonometric Function3/1, Trigonometric Function1/1, Add/2
  angle/1 -> K1/1
  Tap_pu/1 -> K4/1
  Udio/1 -> Product3/1, Divide1/1, Product4/1
  Product/1 -> Divide1/2
  K/1 -> Product/2
  c/1 -> K/1
  K3/1 -> Product2/1
  K4/1 -> Product/1, Product3/2, Product4/2
  Product3/1 -> K5/1
  K5/1 -> P_q/1
  [I_d] -> Product4/3
  Product4/1 -> K6/1
  K6/1 -> P_d/1
